simulink model "Testbed_simulation_FA23"  (R2019a)
settings: Solver=ode45  StartTime=0.0  StopTime=10  FixedStep=5e-7  MaxStep=0.01  RelTol=1e-3  EnableMultiTasking=on
undefined symbols (not defined in the file or in its folder): A, Area, B, beta, c, C, CSArea, d, D, dx, fric, G, kd, L, Pa0, Pgain, piston_mass, ps, pt, V_A, V_B, xdot0
libraries: simulink x8
settings Model: Creator=vnatara2  LastModifiedBy=OyunaA
settings DataIOCC: SaveFormat=Array  SignalLoggingSaveFormat=ModelDataLogs  SaveOutput=off  SaveTime=off  ReturnWorkspaceOutputs=off  TimeSaveName=tout2
settings OptimizationCC: ExpressionDepthLimit=2147483647  InitFltsAndDblsToZero=on  LifeSpan=inf
settings DebuggingCC: SaveWithParameterizedLinksMsg=none  UnderspecifiedInitializationDetection=Classic  MergeDetectMultiDrivingBlocksExec=none  SolverPrmCheckMsg=warning  FcnCallInpInsideContextMsg=warning  AllowSymbolicDim=off  StateNameClashWarn=warning  PregeneratedLibrarySubsystemCodeDiagnostic=none  SFUnexpectedBacktrackingDiag=warning  SFNoUnconditionalDefaultTransitionDiag=warning  SFExecutionAtInitializationDiag=none  ArithmeticOperatorsInVariantConditions=warning
settings HardwareCC: ProdBitPerPointer=32  ProdBitPerSizeT=32  ProdBitPerPtrDiffT=32  ProdLargestAtomicFloat=None  ProdIntDivRoundTo=Undefined  ProdEndianess=Unspecified  ProdWordSize=32  ProdHWDeviceType=32-bit Generic
settings ModelReferenceCC: PropagateSignalLabelsOutOfModel=off
settings SFSimCC: SimUseLocalCustomCode=off
settings RTWCC: RTWUseLocalCustomCode=off
settings CodeAppCC: StateflowObjectComments=on
settings GRTTargetCC: TargetFcnLib=ansi_tfl_tmw.mat  TargetLangStandard=C89/C90 (ANSI)  GeneratePreprocessorConditionals=Disable all  CombineOutputUpdateFcns=off  GRTInterface=on
settings ConfigComp: CovMetricSettings=dw  CovHtmlReporting=on  CovSaveCumulativeToWorkspaceVar=on  CovSaveSingleToWorkspaceVar=on  CovExternalEMLEnable=off  CovSFcnEnable=off

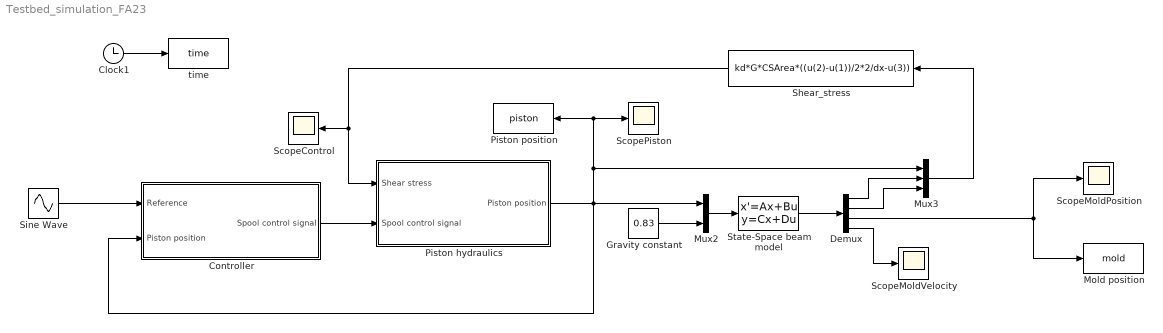
== system Testbed_simulation_FA23 ==
  Clock1 : Clock
  Controller : Subsystem
  Demux : Demux
  Gravity constant : Constant  Value=0.83
  Mold position : ToWorkspace  VariableName=mold  SampleTime=0.002
      settings: MaxDataPoints=1250
  Mux2 : Mux  Inputs=2
  Mux3 : Mux  Inputs=3
  Piston hydraulics : Subsystem
  Piston position : ToWorkspace  VariableName=piston  SampleTime=0.002
      settings: MaxDataPoints=1250
  ScopeControl : Scope
  ScopeMoldPosition : Scope
  ScopeMoldVelocity : Scope
  ScopePiston : Scope
  Shear_stress : Fcn  Expr=kd*G*CSArea*((u(2)-u(1))/2*2/dx-u(3))
  Sine Wave : Sin  Amplitude=3.05/1000  Frequency=2*pi*4.6  SampleTime=0
  State-Space beam model : StateSpace  A=A  B=B  C=C  D=D  InitialCondition=0
  time : ToWorkspace  VariableName=time  SampleTime=0.002
      settings: MaxDataPoints=1250
  wires:
  Piston hydraulics/1(Piston position) -> Mux2/1, ScopePiston/1, Piston position/1, Mux3/1, Controller/2(Piston position)
  Mux2/1 -> State-Space beam model/1
  Gravity constant/1 -> Mux2/2
  Mux3/1 -> Shear_stress/1
  Clock1/1 -> time/1
  State-Space beam model/1 -> Demux/1
  Demux/1 -> Mux3/2
  Demux/2 -> Mux3/3
  Demux/3 -> Mold position/1, ScopeMoldPosition/1
  Demux/4 -> ScopeMoldVelocity/1
  Shear_stress/1 -> Piston hydraulics/1(Shear stress), ScopeControl/1
  Sine Wave/1 -> Controller/1(Reference)
  Controller/1(Spool control signal) -> Piston hydraulics/2(Spool control signal)

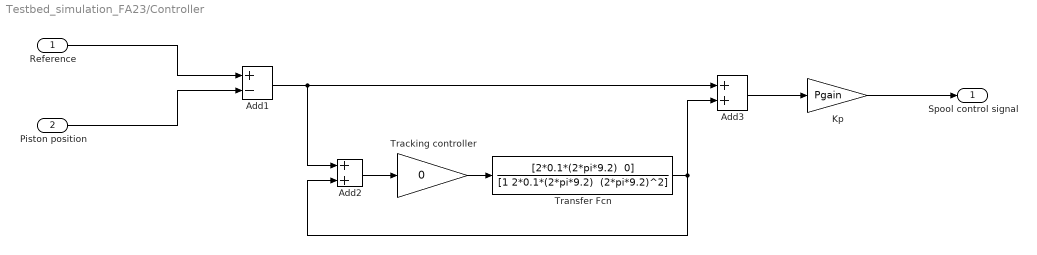
== system Testbed_simulation_FA23/Controller ==
  Reference : Inport
  Piston position : Inport  Port=2
  Add1 : Sum  Inputs=+-
  Add2 : Sum
  Add3 : Sum
  Kp : Gain  Gain=Pgain
  Tracking controller : Gain  Gain=0
  Transfer Fcn : TransferFcn  Numerator="[2*0.1*(2*pi*9.2)  0]"  Denominator="[1 2*0.1*(2*pi*9.2)  (2*pi*9.2)^2]"
  Spool control signal : Outport
  wires:
  Piston position/1 -> Add1/2
  Add1/1 -> Add2/1, Add3/1
  Add2/1 -> Tracking controller/1
  Tracking controller/1 -> Transfer Fcn/1
  Transfer Fcn/1 -> Add2/2, Add3/2
  Add3/1 -> Kp/1
  Kp/1 -> Spool control signal/1
  Reference/1 -> Add1/1

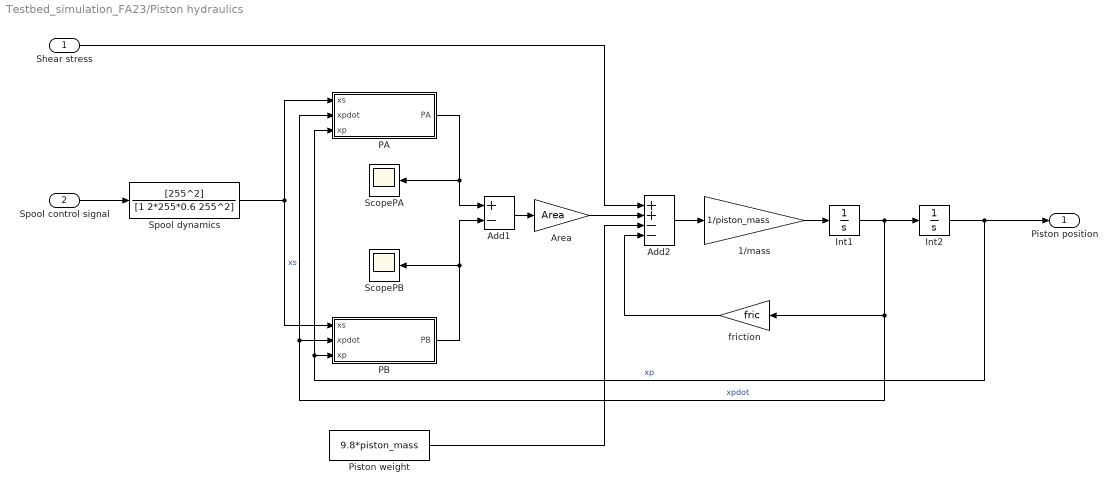
== system Testbed_simulation_FA23/Piston hydraulics ==
  Shear stress : Inport
  Spool control signal : Inport  Port=2
  1/mass : Gain  Gain=1/piston_mass
  Add1 : Sum  Inputs=+-
  Add2 : Sum  Inputs=++--
  Area : Gain  Gain=Area
  Int1 : Integrator  InitialCondition=xdot0
  Int2 : Integrator  InitialCondition=xdot0
  PA : Subsystem
  PB : Subsystem
  Piston weight : Constant  Value=9.8*piston_mass
  ScopePA : Scope
  ScopePB : Scope
  Spool dynamics : TransferFcn  Numerator=[255^2]  Denominator=[1 2*255*0.6 255^2]
  friction : Gain  Gain=fric
  Piston position : Outport
  wires:
  Spool dynamics/1 -> PA/1(xs), PB/1(xs)  "xs"
  PA/1(PA) -> Add1/1, ScopePA/1
  PB/1(PB) -> Add1/2, ScopePB/1
  Add1/1 -> Area/1
  Add2/1 -> 1/mass/1
  Piston weight/1 -> Add2/3
  1/mass/1 -> Int1/1
  Int1/1 -> Int2/1, friction/1, PA/2(xpdot), PB/2(xpdot)  "xpdot"
  Int2/1 -> Piston position/1, PB/3(xp), PA/3(xp)  "xp"
  friction/1 -> Add2/4
  Shear stress/1 -> Add2/1
  Spool control signal/1 -> Spool dynamics/1
  Area/1 -> Add2/2

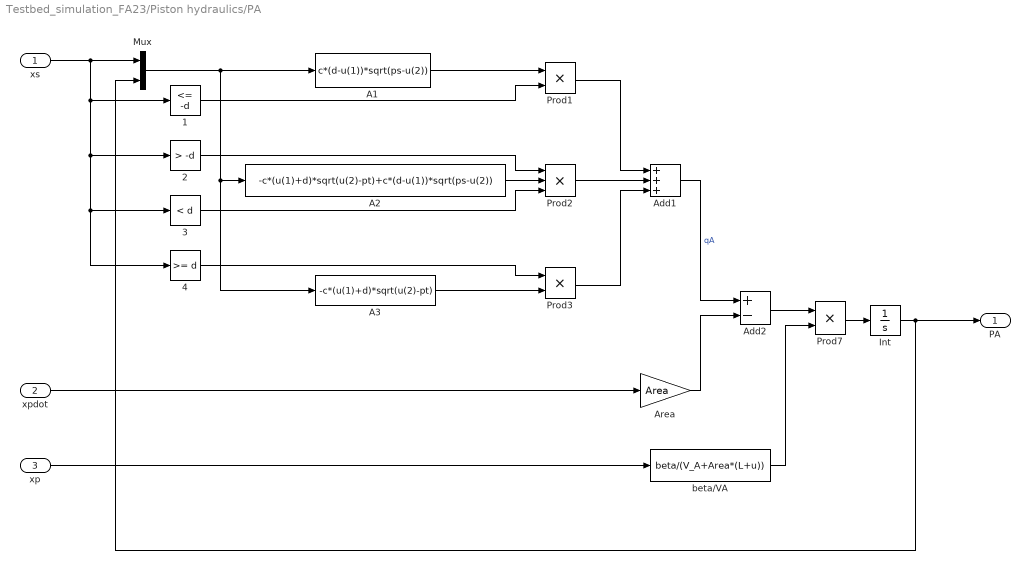
== system Testbed_simulation_FA23/Piston hydraulics/PA ==
  xs : Inport
  xpdot : Inport  Port=2
  xp : Inport  Port=3
  1 : simulink/Logic and Bit Operations/Compare To Constant  relop=<=  const=-d  OutDataTypeStr=uint8  ZeroCross=off
  2 : simulink/Logic and Bit Operations/Compare To Constant  relop=>  const=-d  OutDataTypeStr=uint8  ZeroCross=off
  3 : simulink/Logic and Bit Operations/Compare To Constant  relop=<  const=d  OutDataTypeStr=uint8  ZeroCross=off
  4 : simulink/Logic and Bit Operations/Compare To Constant  relop=>=  const=d  OutDataTypeStr=uint8  ZeroCross=off
  A1 : Fcn  Expr=c*(d-u(1))*sqrt(ps-u(2))
  A2 : Fcn  Expr=-c*(u(1)+d)*sqrt(u(2)-pt)+c*(d-u(1))*sqrt(ps-u(2))
  A3 : Fcn  Expr=-c*(u(1)+d)*sqrt(u(2)-pt)
  Add1 : Sum  Inputs=+++
  Add2 : Sum  Inputs=+-
  Area : Gain  Gain=Area
  Int : Integrator  InitialCondition=Pa0  LimitOutput=on  UpperSaturationLimit=ps  LowerSaturationLimit=pt
  Mux : Mux  Inputs=2
  Prod1 : Product  RndMeth=Zero
  Prod2 : Product  Inputs=3  RndMeth=Zero
  Prod3 : Product  RndMeth=Zero
  Prod7 : Product  RndMeth=Zero
  beta/VA : Fcn  Expr=beta/(V_A+Area*(L+u))
  PA : Outport
  wires:
  A3/1 -> Prod3/2
  2/1 -> Prod2/1
  Prod2/1 -> Add1/2
  Prod3/1 -> Add1/3
  Mux/1 -> A1/1, A2/1, A3/1
  A1/1 -> Prod1/1
  1/1 -> Prod1/2
  A2/1 -> Prod2/2
  3/1 -> Prod2/3
  Prod1/1 -> Add1/1
  4/1 -> Prod3/1
  xs/1 -> Mux/1, 1/1, 2/1, 3/1, 4/1
  Add1/1 -> Add2/1  "qA"
  xpdot/1 -> Area/1
  Area/1 -> Add2/2
  Add2/1 -> Prod7/1
  xp/1 -> beta/VA/1
  beta/VA/1 -> Prod7/2
  Prod7/1 -> Int/1
  Int/1 -> Mux/2, PA/1

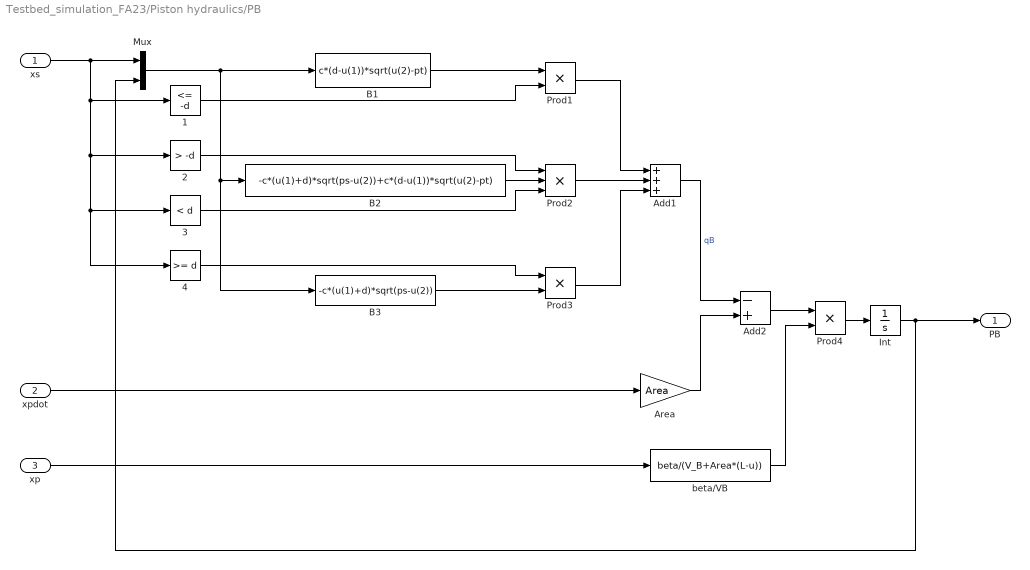
== system Testbed_simulation_FA23/Piston hydraulics/PB ==
  xs : Inport
  xpdot : Inport  Port=2
  xp : Inport  Port=3
  1 : simulink/Logic and Bit Operations/Compare To Constant  relop=<=  const=-d  OutDataTypeStr=uint8  ZeroCross=off
  2 : simulink/Logic and Bit Operations/Compare To Constant  relop=>  const=-d  OutDataTypeStr=uint8  ZeroCross=off
  3 : simulink/Logic and Bit Operations/Compare To Constant  relop=<  const=d  OutDataTypeStr=uint8  ZeroCross=off
  4 : simulink/Logic and Bit Operations/Compare To Constant  relop=>=  const=d  OutDataTypeStr=uint8  ZeroCross=off
  Add1 : Sum  Inputs=+++
  Add2 : Sum  Inputs=-+
  Area : Gain  Gain=Area
  B1 : Fcn  Expr=c*(d-u(1))*sqrt(u(2)-pt)
  B2 : Fcn  Expr=-c*(u(1)+d)*sqrt(ps-u(2))+c*(d-u(1))*sqrt(u(2)-pt)
  B3 : Fcn  Expr=-c*(u(1)+d)*sqrt(ps-u(2))
  Int : Integrator  InitialCondition=Pa0  LimitOutput=on  UpperSaturationLimit=ps  LowerSaturationLimit=pt
  Mux : Mux  Inputs=2
  Prod1 : Product  RndMeth=Zero
  Prod2 : Product  Inputs=3  RndMeth=Zero
  Prod3 : Product  RndMeth=Zero
  Prod4 : Product  RndMeth=Zero
  beta/VB : Fcn  Expr=beta/(V_B+Area*(L-u))
  PB : Outport
  wires:
  B3/1 -> Prod3/2
  2/1 -> Prod2/1
  Prod2/1 -> Add1/2
  Prod3/1 -> Add1/3
  Mux/1 -> B1/1, B2/1, B3/1
  B1/1 -> Prod1/1
  1/1 -> Prod1/2
  B2/1 -> Prod2/2
  3/1 -> Prod2/3
  Prod1/1 -> Add1/1
  4/1 -> Prod3/1
  xs/1 -> Mux/1, 1/1, 2/1, 3/1, 4/1
  Add1/1 -> Add2/1  "qB"
  xpdot/1 -> Area/1
  Area/1 -> Add2/2
  Add2/1 -> Prod4/1
  xp/1 -> beta/VB/1
  beta/VB/1 -> Prod4/2
  Prod4/1 -> Int/1
  Int/1 -> Mux/2, PB/1
